simulink model "tetheredKiteModel"  (R2019a)
settings: Solver=VariableStepAuto  StartTime=0.0  StopTime=20  RelTol=1e-3
undefined symbols (not defined in the file or in its folder): magnitude
libraries: angleBtw2Vecs_ul x5, accelerationCalculator_ul x5, vrlib x4
(part 2 of 2)

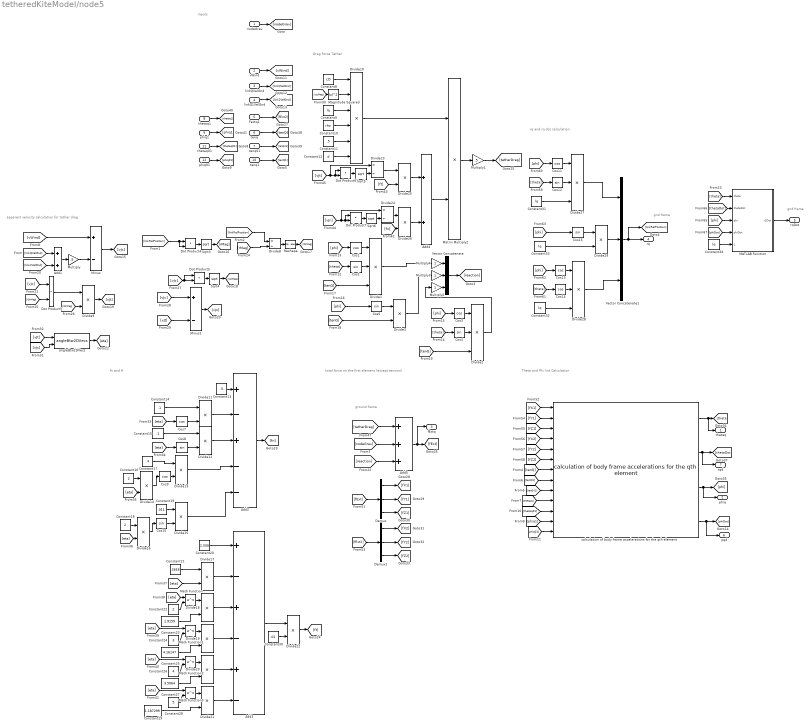
== system tetheredKiteModel/node5  ==
  note: gnd frame
  note: fn and ft
  note: gnd frame
  note: inputs
  note: apparent velocity calculation for tether drag
  note: ground frame
  note: rq and rq dot calculation
  note: Theta and Phi link Calculation
  note: total force on the first element
      |  (except tension)
  note: Drag Force Tether
  nodeGrav : Inport
  vWind : Inport  Port=2
  "linkQVelGnd " : Inport  Port=3
  linkQ1VelGnd : Inport  Port=4
  Fextq1 : Inport  Port=5
  "tenq " : Inport  Port=6
  tenq01 : Inport  Port=7
  "thetaq1 " : Inport  Port=8
  phiq1 : Inport  Port=9
  tenq1 : Inport  Port=10
  thetaq01 : Inport  Port=11
  phiq01 : Inport  Port=12
  Add1 : Sum
  Add2 : Sum  Inputs=+-+--
  Add3 : Sum  Inputs=+-+-+-
  Add4 : Sum
  Add5 : Sum  Inputs=+++
  Constant10 : Constant  Value=rho
  Constant11 : Constant  Value=.5
  Constant12 : Constant  Value=d
  Constant13 : Constant  Value=.5
  Constant14 : Constant  Value=.1
  Constant15 : Constant  Value=.1
  Constant16 : Constant  Value=2
  Constant17 : Constant  Value=.4
  Constant18 : Constant  Value=2
  Constant19 : Constant  Value=.011
  Constant20 : Constant  Value=2.008
  Constant21 : Constant  Value=.3858
  Constant22 : Constant  Value=2
  Constant23 : Constant  Value=1.9159
  Constant24 : Constant  Value=3
  Constant25 : Constant  Value=4.16147
  Constant26 : Constant  Value=4
  Constant27 : Constant  Value=3.5064
  Constant28 : Constant  Value=5
  Constant29 : Constant  Value=1.187299
  Constant30 : Constant  Value=.01
  Constant{9,31..34} (5 alike) : Constant  Value=lq
  Constant8 : Constant  Value=cD
  Cos{1,3,7,9,11,13..14} (7 alike) : Trigonometry  Operator=cos
  Cos{2,4..5,8,10,12,15} (7 alike) : Trigonometry
  Demux : Demux  Outputs=3
  Demux1 : Demux  Outputs=3
  Divide{1..2,27..28} (4 alike) : Product  Inputs=***
  Divide10 : Product  Inputs=******
  Divide{3,9,11..22,25..26,29} (17 alike) : Product  Inputs=**
  Divide23 : Product  Inputs=*/
  Divide24 : Product  Inputs=*/
  Divide8 : Product  Inputs=*/
  Dot Product{3..7} (5 alike) : DotProduct  InputSameDT=on  OutDataTypeStr=Inherit: Inherit via internal rule
  MATLAB Function : MATLAB Function  TreatAsAtomicUnit=on
  Magnitude Squared : Math  Operator=magnitude^2  SaturateOnIntegerOverflow=on
  Math Function{,1..3} (4 alike) : Math  Operator=pow  SaturateOnIntegerOverflow=on
  Matrix Multiply2 : Product
  Minus : Sum  Inputs=+-
  Minus1 : Sum  Inputs=+-
  Multiply : Gain  Gain=.5
  Multiply1 : Gain  Gain=.5
  Multiply2 : Gain
  Multiply3 : Gain
  Multiply4 : Gain
  Reshape : Reshape  OutputDimensionality=Column vector (2-D)
  Sqrt{3..6} (4 alike) : Sqrt  SaturateOnIntegerOverflow=on
  Vector Concatenate : Concatenate  NumInputs=3
  Vector Concatenate1 : Concatenate  NumInputs=3
  angleBtw2DVecs : angleBtw2Vecs_ul/angleBtw2DVecs  SystemSampleTime=-1
  calculation of body frame accelerations for the qth element : accelerationCalculator_ul/calculation of body frame accelerations for the qth element  mj=1000*200*pi*.0005*.0005  mj1=1000*200*pi*.0005*.0005  L=200
  thetaq : Outport
  phiq : Outport  Port=2
  fExtq : Outport  Port=3
  "rq " : Outport  Port=4
  rqDot : Outport  Port=5
  pqd : Outport  Port=6
  tqd : Outport  Port=7
  wires:
  Cos14/1 -> Divide28/2
  Constant32/1 -> Divide28/3
  Cos15/1 -> Divide29/1
  Constant34/1 -> MATLAB Function/5(L)
  Demux/3 -> [fZ1]
  Divide16/1 -> Cos10/1
  Cos10/1 -> Divide15/2
  Constant18/1 -> Divide16/1
  Divide21/1 -> Add3/6
  Constant21/1 -> Divide17/1
  [fZ1] -> calculation of body frame accelerations for the qth element/3
  tenq01/1 -> [tenQ01]
  [phi] -> Cos15/1
  MATLAB Function/1(r1Dot) -> rqDot/1
  [vJc] -> angleBtw2DVecs/2
  Magnitude Squared/1 -> Divide10/2
  [phi] -> Cos11/1
  [fExt] -> Demux/1
  [phiq01] -> calculation of body frame accelerations for the qth element/13
  Demux1/2 -> [fY2]
  Constant14/1 -> Divide11/1
  Demux1/1 -> [fX2]
  [eta] -> Divide17/2
  [phi] -> MATLAB Function/3(phi)
  Divide22/1 -> [ft]
  Divide15/1 -> Add2/5
  Constant11/1 -> Divide10/5
  Constant12/1 -> Divide10/6
  Divide19/1 -> Add3/4
  Cos12/1 -> Divide27/2
  [tetherDrag] -> Add5/1
  [thetaDot] -> MATLAB Function/2(thetaDot)
  [vJc] -> Dot Product5/1, Dot Product5/2
  [rMag] -> Divide8/2
  [eta] -> Cos8/1
  Constant15/1 -> Divide12/1
  Sqrt4/1 -> [vJcMag]
  Add3/1 -> Divide22/1
  Divide27/1 -> Vector Concatenate1/1
  Cos13/1 -> Divide28/1
  Sqrt3/1 -> [rMag]
  Add4/1 -> Matrix Multiply2/2
  Cos7/1 -> Divide11/2
  Multiply/1 -> Minus/2
  Vector Concatenate1/1 -> [linkRelPosition], "rq "/1
  Divide11/1 -> Add2/2
  Dot Product5/1 -> Sqrt4/1
  [vJcMag] -> Magnitude Squared/1
  Minus/1 -> [vJc]
  [theta] -> Cos14/1
  Constant33/1 -> Divide29/2
  [theta] -> MATLAB Function/1(theta)
  [rDrMag] -> Divide9/2
  Minus1/1 -> [vJn]
  Divide8/1 -> Reshape/1
  Dot Product3/1 -> Divide9/1
  [vJt] -> angleBtw2DVecs/1
  nodeGrav/1 -> [nodeGrav]
  [fX2] -> calculation of body frame accelerations for the qth element/4
  Constant23/1 -> Divide18/2
  [fY2] -> calculation of body frame accelerations for the qth element/5
  [fZ2] -> calculation of body frame accelerations for the qth element/6
  Divide29/1 -> Vector Concatenate1/2
  [vJc] -> Dot Product3/1
  Divide18/1 -> Add3/3
  [phi] -> Cos13/1
  Constant10/1 -> Divide10/4
  Constant8/1 -> Divide10/1
  [eta] -> Cos7/1
  Constant9/1 -> Divide10/3
  Divide17/1 -> Add3/2
  Dot Product4/1 -> Sqrt3/1
  Constant19/1 -> Divide15/1
  Add2/1 -> [fn]
  [vJt] -> Divide23/1, Dot Product6/1, Dot Product6/2
  Add5/1 -> fExtq/1, [fExt]
  Constant13/1 -> Add2/1
  Dot Product6/1 -> Sqrt5/1
  Constant26/1 -> Math Function2/2
  [vWind] -> Minus/1
  [vJc] -> Minus1/1
  Math Function2/1 -> Divide20/1
  [eta] -> Math Function2/1
  Constant27/1 -> Divide20/2
  Fextq1/1 -> [fExt2]
  vWind/1 -> [vWind]
  [rDrMag] -> Dot Product3/2
  [phiDot] -> MATLAB Function/4(phiDot)
  Demux/2 -> [fY1]
  Divide23/1 -> Divide25/1
  Divide26/1 -> Add4/2
  [eta] -> Divide16/2
  Constant30/1 -> Divide22/2
  Divide25/1 -> Add4/1
  Divide9/1 -> [vJt]
  Constant24/1 -> Math Function1/2
  Math Function1/1 -> Divide19/1
  Sqrt6/1 -> Divide24/2
  Demux1/3 -> [fZ2]
  Add1/1 -> Multiply/1
  [link2VelGnd] -> Add1/2
  [fX1] -> calculation of body frame accelerations for the qth element/1
  [ft] -> Divide25/2
  Constant20/1 -> Add3/1
  Divide20/1 -> Add3/5
  [thetaq1] -> calculation of body frame accelerations for the qth element/10
  "thetaq1 "/1 -> [thetaq1]
  [linkRelPosition] -> Dot Product4/2, Dot Product4/1
  [tenQ01] -> calculation of body frame accelerations for the qth element/9
  phiq1/1 -> [phiq1]
  [eta] -> Math Function3/1
  Cos8/1 -> Divide12/2
  Constant25/1 -> Divide19/2
  angleBtw2DVecs/1 -> [eta]
  Constant28/1 -> Math Function3/2
  [eta] -> Divide14/2
  Math Function3/1 -> Divide21/1
  linkQ1VelGnd/1 -> [link2VelGnd]
  Constant29/1 -> Divide21/2
  Divide24/1 -> Divide26/1
  [vJn] -> Divide24/1, Dot Product7/1, Dot Product7/2
  [tenQ] -> calculation of body frame accelerations for the qth element/7
  Constant16/1 -> Divide14/1
  Demux/1 -> [fX1]
  [eta] -> Math Function/1
  Constant17/1 -> Divide13/1
  [vJt] -> Minus1/2
  [linkRelPosition] -> Divide8/1
  Divide10/1 -> Matrix Multiply2/1
  [eta] -> Math Function1/1
  Matrix Multiply2/1 -> Multiply1/1
  Divide28/1 -> Vector Concatenate1/3
  [fY1] -> calculation of body frame accelerations for the qth element/2
  "linkQVelGnd "/1 -> [linkQVelGnd]
  [theta] -> Cos12/1
  Constant31/1 -> Divide27/3
  Sqrt5/1 -> Divide23/2
  [fn] -> Divide26/2
  Math Function/1 -> Divide18/1
  Divide13/1 -> Add2/4
  "tenq "/1 -> [tenQ]
  [nodeGrav] -> Add5/2
  Divide14/1 -> Cos9/1
  Constant22/1 -> Math Function/2
  Divide12/1 -> Add2/3
  [thetaq01] -> calculation of body frame accelerations for the qth element/11
  Multiply1/1 -> [tetherDrag]
  [tenQ1] -> calculation of body frame accelerations for the qth element/8
  Dot Product7/1 -> Sqrt6/1
  Cos11/1 -> Divide27/1
  [fExt2] -> Demux1/1
  [linkQVelGnd] -> Add1/1
  Cos9/1 -> Divide13/2
  tenq1/1 -> [tenQ1]
  thetaq01/1 -> [thetaq01]
  phiq01/1 -> [phiq01]
  [phiq1] -> calculation of body frame accelerations for the qth element/12
  Divide1/1 -> Multiply4/1
  Cos2/1 -> Divide1/2
  [phi] -> Cos1/1
  [tenQ] -> Divide3/2
  Cos5/1 -> Divide3/1
  [phi] -> Cos3/1
  [tenQ] -> Divide2/3
  Cos1/1 -> Divide1/1
  Cos3/1 -> Divide2/1
  [theta] -> Cos4/1
  Divide2/1 -> Multiply2/1
  [theta] -> Cos2/1
  Cos4/1 -> Divide2/2
  [phi] -> Cos5/1
  [tenQ] -> Divide1/3
  Multiply2/1 -> Vector Concatenate/3
  Multiply3/1 -> Vector Concatenate/2
  Multiply4/1 -> Vector Concatenate/1
  Divide3/1 -> Multiply3/1
  Vector Concatenate/1 -> [reaction]
  [reaction] -> Add5/3
  Reshape/1 -> [rDrMag]
  calculation of body frame accelerations for the qth element/4 -> pqd/1, [phiDot]
  calculation of body frame accelerations for the qth element/1 -> thetaq/1, [theta]
  calculation of body frame accelerations for the qth element/2 -> tqd/1, [thetaDot]
  calculation of body frame accelerations for the qth element/3 -> phiq/1, [phi]

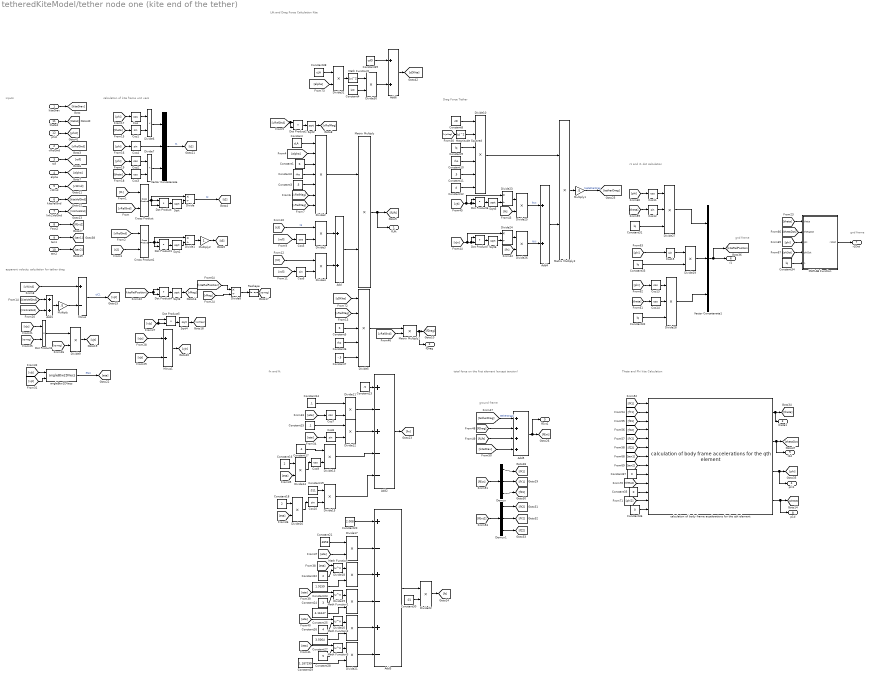
== system tetheredKiteModel/tether node one (kite end of the tether)  ==
  note: gnd frame
  note: r1 and r1 dot calculation
  note: Theta and Phi kite Calculation
  note: ground frame
  note: total force on the first element
      |  (except tension)
  note: fn and ft
  note: Drag Force Tether
  note: apparent velocity calculation for tether drag
  note: Lift and Drag Force Calculation Kite
  note: calculation of kite frame unit vecs
  note: inputs
  note: gnd frame
  kiteGrav : Inport
  vRelGnd : Inport  Port=2
  roll : Inport  Port=3
  alpha : Inport  Port=4
  vWind : Inport  Port=5
  "kiteVelGnd " : Inport  Port=6
  link2VelGnd : Inport  Port=7
  Fext2 : Inport  Port=8
  "ten1 " : Inport  Port=9
  ten2 : Inport  Port=10
  "theta2 " : Inport  Port=11
  phi2 : Inport  Port=12
  Add{,1,4,6} (4 alike) : Sum
  Add2 : Sum  Inputs=+-+--
  Add3 : Sum  Inputs=+-+-+-
  Add5 : Sum  Inputs=++++
  Constant : Constant  Value=cLA
  Constant1 : Constant  Value=S
  Constant10 : Constant  Value=rho
  Constant11 : Constant  Value=.5
  Constant12 : Constant  Value=d
  Constant13 : Constant  Value=.5
  Constant14 : Constant  Value=.1
  Constant15 : Constant  Value=.1
  Constant16 : Constant  Value=2
  Constant17 : Constant  Value=.4
  Constant18 : Constant  Value=2
  Constant19 : Constant  Value=.011
  Constant2 : Constant  Value=rho
  Constant20 : Constant  Value=2.008
  Constant21 : Constant  Value=.3858
  Constant22 : Constant  Value=2
  Constant23 : Constant  Value=1.9159
  Constant24 : Constant  Value=3
  Constant25 : Constant  Value=4.16147
  Constant26 : Constant  Value=4
  Constant27 : Constant  Value=3.5064
  Constant28 : Constant  Value=5
  Constant29 : Constant  Value=1.187299
  Constant3 : Constant  Value=.5
  Constant30 : Constant  Value=.01
  Constant{9,31..34} (5 alike) : Constant  Value=lq
  Constant35 : Constant  Value=0
  Constant36 : Constant  Value=0
  Constant37 : Constant  Value=0
  Constant38 : Constant  Value=cLA
  Constant39 : Constant  Value=cdO
  Constant4 : Constant  Value=kO
  Constant5 : Constant  Value=S
  Constant6 : Constant  Value=rho
  Constant7 : Constant  Value=-.5
  Constant8 : Constant  Value=cD
  Cos{,2..3,5,7,9,11,13..14} (9 alike) : Trigonometry  Operator=cos
  Cos{1,4,6,8,10,12,15} (7 alike) : Trigonometry
  Cross Product : vrlib/Utilities/Cross Product
      settings: SourceProductName=Simulink
  Cross Product1 : vrlib/Utilities/Cross Product
      settings: SourceProductName=Simulink
  Demux : Demux  Outputs=3
  Demux1 : Demux  Outputs=3
  Divide{,1,8,23..24} (5 alike) : Product  Inputs=*/
  Divide10 : Product  Inputs=******
  Divide{3..4,6..7,9,11..22,25..26,29..31} (22 alike) : Product  Inputs=**
  Divide2 : Product  Inputs=*******
  Divide27 : Product  Inputs=***
  Divide28 : Product  Inputs=***
  Divide5 : Product  Inputs=*****
  Dot Product{,1..7} (8 alike) : DotProduct  InputSameDT=on  OutDataTypeStr=Inherit: Inherit via internal rule
  MATLAB Function : MATLAB Function  TreatAsAtomicUnit=on
  Magnitude Squared : Math  Operator=magnitude^2  SaturateOnIntegerOverflow=on
  Math Function{,1..3} (4 alike) : Math  Operator=pow  SaturateOnIntegerOverflow=on
  Math Function5 : Math  Operator=magnitude^2  SaturateOnIntegerOverflow=on
  Matrix Multiply : Product
  Matrix Multiply1 : Product
  Matrix Multiply2 : Product
  Minus : Sum  Inputs=+-
  Minus1 : Sum  Inputs=+-
  Multiply : Gain  Gain=.5
  Multiply1 : Gain  Gain=.5
  Multiply2 : Gain
  Reshape : Reshape  OutputDimensionality=Column vector (2-D)
  Sqrt{,1..6} (7 alike) : Sqrt  SaturateOnIntegerOverflow=on
  Vector Concatenate : Concatenate  NumInputs=3
  Vector Concatenate1 : Concatenate  NumInputs=3
  angleBtw2DVecs : angleBtw2Vecs_ul/angleBtw2DVecs  SystemSampleTime=-1
  calculation of body frame accelerations for the qth element : accelerationCalculator_ul/calculation of body frame accelerations for the qth element  mj=20 + .5*1000*200*pi*.0005*.0005  mj1=1000*200*pi*.0005*.0005  L=200
  "fLift " : Outport
  "fDrag " : Outport  Port=2
  theta1 : Outport  Port=3
  phi1 : Outport  Port=4
  fExt1 : Outport  Port=5
  "r1 " : Outport  Port=6
  r1Dot : Outport  Port=7
  p1d : Outport  Port=8
  t1d : Outport  Port=9
  wires:
  Cos3/1 -> Divide7/2
  [phi] -> Cos4/1
  [phi] -> Cos2/1
  Cos/1 -> Divide6/1
  Cos4/1 -> Vector Concatenate/2
  [theta] -> Cos3/1
  [theta] -> Cos1/1
  Vector Concatenate/1 -> [t1]  "t1"
  Divide7/1 -> Vector Concatenate/3
  Cos2/1 -> Divide7/1
  Cos1/1 -> Divide6/2
  [phi] -> Cos/1
  Divide6/1 -> Vector Concatenate/1
  kiteGrav/1 -> [kiteGrav]
  vRelGnd/1 -> [vRelGnd]
  Cross Product/1 -> Dot Product/2, Dot Product/1, Divide/1
  Dot Product/1 -> Sqrt/1
  Sqrt/1 -> Divide/2
  Divide/1 -> [t2]  "t2"
  [vRelGnd] -> Cross Product/2
  [t1] -> Cross Product/1
  [vRelGnd] -> Cross Product1/1
  [t2] -> Cross Product1/2
  Sqrt1/1 -> Divide1/2
  Cross Product1/1 -> Dot Product1/2, Dot Product1/1, Divide1/1
  Dot Product1/1 -> Sqrt1/1
  Divide1/1 -> Multiply2/1
  roll/1 -> [roll]
  alpha/1 -> [alpha]
  Constant/1 -> Divide2/1
  [alpha] -> Divide2/2
  Constant1/1 -> Divide2/3
  Constant2/1 -> Divide2/4
  Constant3/1 -> Divide2/5
  [vRelGnd] -> Dot Product2/2, Dot Product2/1
  Dot Product2/1 -> Sqrt2/1
  Sqrt2/1 -> [vRelMag]
  [vRelMag] -> Divide2/6
  [vRelMag] -> Divide2/7
  Cos5/1 -> Divide3/2
  [roll] -> Cos5/1
  [t3] -> Divide3/1  "t3"
  [roll] -> Cos6/1
  [t2] -> Divide4/1
  Cos6/1 -> Divide4/2
  Divide3/1 -> Add/1
  Divide4/1 -> Add/2
  Add/1 -> Matrix Multiply/2
  Divide2/1 -> Matrix Multiply/1
  Matrix Multiply/1 -> "fLift "/1, [fLift]
  Constant5/1 -> Divide5/3
  [cDKite] -> Divide5/1
  Constant6/1 -> Divide5/4
  [vRelMag] -> Divide5/2
  Constant7/1 -> Divide5/5
  vWind/1 -> [vWind]
  "kiteVelGnd "/1 -> [kiteVelGnd]
  link2VelGnd/1 -> [link2VelGnd]
  [kiteVelGnd] -> Add1/1
  [link2VelGnd] -> Add1/2
  Add1/1 -> Multiply/1
  [vWind] -> Minus/1
  Multiply/1 -> Minus/2
  Minus/1 -> [vJc]  "vJC1"
  [vJc] -> Dot Product3/1
  [rDrMag] -> Dot Product3/2
  [kiteRelPosition] -> Dot Product4/1, Dot Product4/2
  Dot Product4/1 -> Sqrt3/1
  Sqrt3/1 -> [rMag]
  [kiteRelPosition] -> Divide8/1
  [rMag] -> Divide8/2
  Divide8/1 -> Reshape/1
  Dot Product3/1 -> Divide9/1
  [rDrMag] -> Divide9/2
  [vJc] -> Dot Product5/1, Dot Product5/2
  Dot Product5/1 -> Sqrt4/1
  Sqrt4/1 -> [vJcMag]
  Divide9/1 -> [vJt]
  [vJc] -> Minus1/1
  [vJt] -> Minus1/2
  Minus1/1 -> [vJn]
  Constant11/1 -> Divide10/5
  Magnitude Squared/1 -> Divide10/2
  Constant8/1 -> Divide10/1
  Constant9/1 -> Divide10/3
  Constant10/1 -> Divide10/4
  Constant12/1 -> Divide10/6
  [vJcMag] -> Magnitude Squared/1
  [vJc] -> angleBtw2DVecs/2
  [vJt] -> angleBtw2DVecs/1
  angleBtw2DVecs/1 -> [eta]  "eta1"
  Constant13/1 -> Add2/1
  Cos7/1 -> Divide11/2
  [eta] -> Cos7/1
  Constant14/1 -> Divide11/1
  Divide11/1 -> Add2/2
  Constant15/1 -> Divide12/1
  Cos8/1 -> Divide12/2
  [eta] -> Cos8/1
  Divide12/1 -> Add2/3
  Divide13/1 -> Add2/4
  Divide14/1 -> Cos9/1
  Cos9/1 -> Divide13/2
  [eta] -> Divide14/2
  Constant16/1 -> Divide14/1
  Constant17/1 -> Divide13/1
  Constant19/1 -> Divide15/1
  Constant18/1 -> Divide16/1
  Cos10/1 -> Divide15/2
  Divide15/1 -> Add2/5
  Divide16/1 -> Cos10/1
  [eta] -> Divide16/2
  Add2/1 -> [fn]
  Constant20/1 -> Add3/1
  Divide17/1 -> Add3/2
  Constant21/1 -> Divide17/1
  [eta] -> Divide17/2
  Divide18/1 -> Add3/3
  Math Function/1 -> Divide18/1
  [eta] -> Math Function/1
  Constant22/1 -> Math Function/2
  Constant23/1 -> Divide18/2
  Constant25/1 -> Divide19/2
  Math Function1/1 -> Divide19/1
  [eta] -> Math Function1/1
  Constant24/1 -> Math Function1/2
  Divide19/1 -> Add3/4
  Constant27/1 -> Divide20/2
  Math Function2/1 -> Divide20/1
  [eta] -> Math Function2/1
  Constant26/1 -> Math Function2/2
  Divide20/1 -> Add3/5
  Divide21/1 -> Add3/6
  Constant28/1 -> Math Function3/2
  Math Function3/1 -> Divide21/1
  [eta] -> Math Function3/1
  Constant29/1 -> Divide21/2
  Add3/1 -> Divide22/1
  Constant30/1 -> Divide22/2
  Divide22/1 -> [ft]
  Dot Product6/1 -> Sqrt5/1
  Dot Product7/1 -> Sqrt6/1
  [vJn] -> Divide24/1, Dot Product7/1, Dot Product7/2
  [vJt] -> Divide23/1, Dot Product6/1, Dot Product6/2
  Sqrt5/1 -> Divide23/2
  Sqrt6/1 -> Divide24/2
  Divide24/1 -> Divide26/1
  Divide5/1 -> Matrix Multiply1/1
  [vRelGnd] -> Matrix Multiply1/2
  Matrix Multiply1/1 -> "fDrag "/1, [fDrag]
  [fn] -> Divide26/2
  Divide23/1 -> Divide25/1
  [ft] -> Divide25/2
  Divide25/1 -> Add4/1  "fnVj"
  Divide26/1 -> Add4/2  "ftVj"
  Add4/1 -> Matrix Multiply2/2
  Divide10/1 -> Matrix Multiply2/1
  Matrix Multiply2/1 -> Multiply1/1
  Multiply1/1 -> [tetherDrag]  "toptetherDrag"
  [kiteGrav] -> Add5/4
  [fLift] -> Add5/3
  [fDrag] -> Add5/2
  [tetherDrag] -> Add5/1  "tetherDrag1"
  Add5/1 -> fExt1/1, [fExt]
  Fext2/1 -> [fExt2]
  [fExt] -> Demux/1
  Demux/1 -> [fX1]
  Demux/2 -> [fY1]
  Demux/3 -> [fZ1]
  Demux1/3 -> [fZ2]
  Demux1/1 -> [fX2]
  Demux1/2 -> [fY2]
  [fExt2] -> Demux1/1
  [fX1] -> calculation of body frame accelerations for the qth element/1
  [fY1] -> calculation of body frame accelerations for the qth element/2
  [fZ1] -> calculation of body frame accelerations for the qth element/3
  [fX2] -> calculation of body frame accelerations for the qth element/4
  [fY2] -> calculation of body frame accelerations for the qth element/5
  [fZ2] -> calculation of body frame accelerations for the qth element/6
  [phi] -> Cos11/1
  [theta] -> Cos12/1
  Cos11/1 -> Divide27/1
  Cos12/1 -> Divide27/2
  Constant31/1 -> Divide27/3
  [phi] -> Cos13/1
  [theta] -> Cos14/1
  Constant32/1 -> Divide28/3
  Cos13/1 -> Divide28/1
  Cos14/1 -> Divide28/2
  [phi] -> Cos15/1
  Cos15/1 -> Divide29/1
  Constant33/1 -> Divide29/2
  Divide29/1 -> Vector Concatenate1/2
  Divide28/1 -> Vector Concatenate1/3
  Divide27/1 -> Vector Concatenate1/1
  Vector Concatenate1/1 -> [kiteRelPosition], "r1 "/1
  [theta] -> MATLAB Function/1(theta)
  [phi] -> MATLAB Function/3(phi)
  Constant34/1 -> MATLAB Function/5(L)
  [phiDot] -> MATLAB Function/4(phiDot)
  [thetaDot] -> MATLAB Function/2(thetaDot)
  MATLAB Function/1(r1Dot) -> r1Dot/1
  Constant36/1 -> calculation of body frame accelerations for the qth element/13
  Constant35/1 -> calculation of body frame accelerations for the qth element/11
  Constant37/1 -> calculation of body frame accelerations for the qth element/9
  "ten1 "/1 -> [ten1]
  ten2/1 -> [ten2]
  [ten2] -> calculation of body frame accelerations for the qth element/8
  [ten1] -> calculation of body frame accelerations for the qth element/7
  "theta2 "/1 -> [theta2]
  phi2/1 -> [phi2]
  [theta2] -> calculation of body frame accelerations for the qth element/10
  [phi2] -> calculation of body frame accelerations for the qth element/12
  Divide31/1 -> Math Function5/1
  [alpha] -> Divide31/2
  Constant38/1 -> Divide31/1
  Math Function5/1 -> Divide30/1
  Constant4/1 -> Divide30/2
  Divide30/1 -> Add6/2
  Constant39/1 -> Add6/1
  Add6/1 -> [cDKite]
  Reshape/1 -> [rDrMag]
  calculation of body frame accelerations for the qth element/1 -> theta1/1, [theta]
  calculation of body frame accelerations for the qth element/2 -> t1d/1, [thetaDot]
  calculation of body frame accelerations for the qth element/3 -> phi1/1, [phi]
  calculation of body frame accelerations for the qth element/4 -> p1d/1, [phiDot]
  Multiply2/1 -> [t3]

== matlab function tetheredKiteModel/node2/MATLAB Function ==
  data: theta input; r1Dot output; thetaDot input; phi input; phiDot input; L input
function r1Dot = fcn(theta,thetaDot,phi,phiDot,L)

r1Dot = zeros(3,1);
r1Dot(1) = -L*phiDot*sin(phi)*sin(theta) + L*thetaDot*cos(phi)*cos(theta);
r1Dot(2) = L*phiDot*cos(phi); 
r1Dot(3) = -L*phiDot*sin(phi)*cos(theta)-L*thetaDot*cos(phi)*sin(theta);

== matlab function tetheredKiteModel/tether node one (kite end of the tether) /MATLAB Function ==
  data: theta input; r1Dot output; thetaDot input; phi input; phiDot input; L input
function r1Dot = fcn(theta,thetaDot,phi,phiDot,L)

r1Dot = zeros(3,1);
r1Dot(1) = -L*phiDot*sin(phi)*sin(theta) + L*thetaDot*cos(phi)*cos(theta);
r1Dot(2) = L*phiDot*cos(phi); 
r1Dot(3) = -L*phiDot*sin(phi)*cos(theta)-L*thetaDot*cos(phi)*sin(theta);

== matlab function tetheredKiteModel/node3/MATLAB Function ==
  data: theta input; r1Dot output; thetaDot input; phi input; phiDot input; L input
function r1Dot = fcn(theta,thetaDot,phi,phiDot,L)

r1Dot = zeros(3,1);
r1Dot(1) = -L*phiDot*sin(phi)*sin(theta) + L*thetaDot*cos(phi)*cos(theta);
r1Dot(2) = L*phiDot*cos(phi); 
r1Dot(3) = -L*phiDot*sin(phi)*cos(theta)-L*thetaDot*cos(phi)*sin(theta);

== matlab function tetheredKiteModel/MATLAB Function2 ==
  data: m1 input; m2 input; m3 input; m4 input; m5 input; ten1 output; t1 input; t2 input; t3 input; t4 input; t5 input; p1 input; p2 input; p3 input; p4 input; p5 input; fx1 input; fx2 input; fx3 input; fx4 input; fx5 input; fx6 input; fy1 input; fy2 input; fy3 input; fy4 input; fy5 input; fy6 input; fz1 input; fz2 input; fz3 input; fz4 input; fz5 input; fz6 input; t1d input; t2d input; t3d input; t4d input; t5d input; p1d input; p2d input; p3d input; p4d input; p5d input; L input; ten2 output; ten3 output; ten4 output; ten5 output
function [ten1,ten2,ten3,ten4,ten5] = fcn(m1,m2,m3,m4,m5,t1,t2,t3,t4,t5,p1,p2,p3,p4,p5,fx1,fx2,fx3,fx4,fx5,fx6,fy1,fy2,fy3,fy4,fy5,fy6,fz1,fz2,fz3,fz4,fz5,fz6,t1d,t2d,t3d,t4d,t5d,p1d,p2d,p3d,p4d,p5d,L)
A = zeros(5,1);
B = zeros(5,5);
A(1) = -L*(cos(p1)^2)*(t1d^2)-L*(p1d^2)-(1/m1)*(fx1*sin(t1)*cos(p1) + fy1*sin(p1)+fz1*cos(t1)*cos(p1)) - (1/m2)*(- fx2*sin(t1)*cos(p1)-fy2*sin(p1)-fz2*cos(t1)*sin(t1));
A(2) = -L*(cos(p2)^2)*(t2d^2)-L*(p2d^2)-(1/m2)*(fx2*sin(t2)*cos(p2) + fy2*sin(p2)+fz2*cos(t2)*cos(p2)) - (1/m3)*(- fx3*sin(t2)*cos(p2)-fy3*sin(p2)-fz3*cos(t2)*sin(t2));
A(3) = -L*(cos(p3)^2)*(t3d^2)-L*(p3d^2)-(1/m3)*(fx3*sin(t3)*cos(p3) + fy3*sin(p3)+fz3*cos(t3)*cos(p3)) - (1/m4)*(- fx4*sin(t3)*cos(p3)-fy4*sin(p3)-fz4*cos(t3)*sin(t3));
A(4) = -L*(cos(p4)^2)*(t4d^2)-L*(p4d^2)-(1/m4)*(fx4*sin(t4)*cos(p4) + fy4*sin(p4)+fz4*cos(t4)*cos(p4)) - (1/m5)*(- fx5*sin(t4)*cos(p4)-fy5*sin(p4)-fz5*cos(t4)*sin(t4));
A(5) = -L*(cos(p5)^2)*(t5d^2)-L*(p5d^2)-(1/m5)*(fx5*sin(t5)*cos(p5) + fy5*sin(p5)+fz5*cos(t5)*cos(p5)) - (1/m5)*(- fx6*sin(t5)*cos(p5)-fy6*sin(p5)-fz6*cos(t5)*sin(t5)); % weird Assumption


B(1,1) = (1/m1)*( -(sin(t1)^2)*(cos(p1)^2) - (sin(p1)^2) - (cos(t1)^2)*(cos(p1)^2)) + (1/m2)*((-sin(t1)^2)*(cos(p1)^2)-(sin(p1)^2) + (cos(t1)^2)*(cos(p1)^2) );
B(1,2) = (1/m2)*(  sin(t1)*cos(p1)*cos(p2)*sin(t2)  + sin(p1)*sin(p2) + cos(t1)*cos(p1)*cos(p2)*cos(t2));
B(1,3) = 0;
B(1,4) = 0;
B(1,5) = 0;

B(2,1) = (1/m2)*(  sin(t2)*cos(p2)*cos(p1)*sin(t1) + sin(p2)*sin(p1) - cos(t2)*cos(p2)*cos(p1)*cos(t1));
B(2,2) = (1/m2)*( -(sin(t2)^2)*(cos(p2)^2) - (sin(p2)^2) - (cos(t2)^2)*(cos(p2)^2)) + (1/m3)*((-sin(t2)^2)*(cos(p2)^2)-(sin(p2)^2) + (cos(t2)^2)*(cos(p2)^2) );
B(2,3) = (1/m3)*(  sin(t2)*cos(p2)*cos(p3)*sin(t3)  + sin(p2)*sin(p3) + cos(t2)*cos(p2)*cos(p3)*cos(t3));
B(2,4) = 0;
B(2,5) = 0;

B(3,1) = 0;
B(3,2) = (1/m3)*(sin(t3)*cos(p3)*cos(p2)*sin(t2) + sin(p3)*sin(p2) - cos(t3)*cos(p3)*cos(p2)*cos(t2));
B(3,3) = (1/m3)*( -(sin(t3)^2)*(cos(p3)^2) - (sin(p3)^2) - (cos(t3)^2)*(cos(p3)^2)) + (1/m4)*((-sin(t3)^2)*(cos(p3)^2)-(sin(p3)^2) + (cos(t3)^2)*(cos(p3)^2) );
B(3,4) = (1/m4)*( sin(t3)*cos(p3)*cos(p4)*sin(t4)  + sin(p3)*sin(p4) + cos(t3)*cos(p3)*cos(p4)*cos(t4));
B(3,5) = 0;

B(4,1) = 0;
B(4,2) = 0;
B(4,3) = (1/m4)*(sin(t4)*cos(p4)*cos(p3)*sin(t3) + sin(p4)*sin(p3) - cos(t4)*cos(p4)*cos(p3)*cos(t3));
B(4,4) = (1/m4)*( -(sin(t4)^2)*(cos(p4)^2) - (sin(p4)^2) - (cos(t4)^2)*(cos(p4)^2)) + (1/m5)*((-sin(t4)^2)*(cos(p4)^2)-(sin(p4)^2) + (cos(t4)^2)*(cos(p4)^2) );
B(4,5) = (1/m5)*( sin(t4)*cos(p4)*cos(p5)*sin(t5)  + sin(p4)*sin(p5) + cos(t4)*cos(p4)*cos(p5)*cos(t5));

B(5,1) = 0;
B(5,2) = 0;
B(5,3) = 0;
B(5,4) = (1/m5)*(sin(t5)*cos(p5)*cos(p4)*sin(t4) + sin(p5)*sin(p4) - cos(t5)*cos(p5)*cos(p4)*cos(t4));
B(5,5) = (1/m5)*( -(sin(t5)^2)*(cos(p5)^2) - (sin(p5)^2) - (cos(t5)^2)*(cos(p5)^2)) + (1/m5)*((-sin(t5)^2)*(cos(p5)^2)-(sin(p5)^2) + (cos(t5)^2)*(cos(p5)^2) );



X = inv(B)*A;

ten1 = X(1); 
ten2 = X(2);
ten3 = X(3);
ten4 = X(4);
ten5 = X(5);
end

== matlab function tetheredKiteModel/node4/MATLAB Function ==
  data: theta input; r1Dot output; thetaDot input; phi input; phiDot input; L input
function r1Dot = fcn(theta,thetaDot,phi,phiDot,L)

r1Dot = zeros(3,1);
r1Dot(1) = -L*phiDot*sin(phi)*sin(theta) + L*thetaDot*cos(phi)*cos(theta);
r1Dot(2) = L*phiDot*cos(phi); 
r1Dot(3) = -L*phiDot*sin(phi)*cos(theta)-L*thetaDot*cos(phi)*sin(theta);

== matlab function tetheredKiteModel/node5 /MATLAB Function ==
  data: theta input; r1Dot output; thetaDot input; phi input; phiDot input; L input
function r1Dot = fcn(theta,thetaDot,phi,phiDot,L)

r1Dot = zeros(3,1);
r1Dot(1) = -L*phiDot*sin(phi)*sin(theta) + L*thetaDot*cos(phi)*cos(theta);
r1Dot(2) = L*phiDot*cos(phi); 
r1Dot(3) = -L*phiDot*sin(phi)*cos(theta)-L*thetaDot*cos(phi)*sin(theta);
